simulink model "simpleSM"  (R2021a)
settings: Solver=ode4  StartTime=0.0  StopTime=10.0  FixedStep=1e-4  RelTol=1e-3
settings Model: Creator=compu  LastModifiedBy=compu

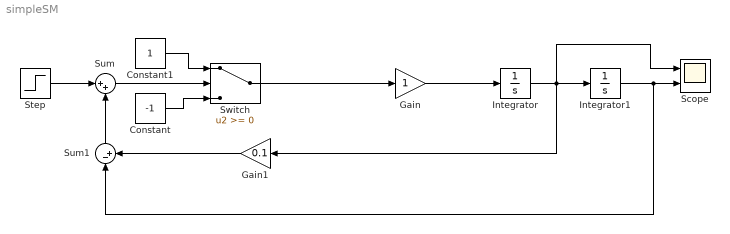
== system simpleSM ==
  Constant : Constant  Value=-1
  Constant1 : Constant
  Gain : Gain
  Gain1 : Gain  Gain=0.1
  Integrator : Integrator
  Integrator1 : Integrator
  Scope : Scope  NumInputPorts=2
  Step : Step  SampleTime=0
  Sum : Sum  Inputs=|++
  Sum1 : Sum  Inputs=|-+
  Switch : Switch  ZeroCross=off
  wires:
  Integrator/1 -> Scope/1, Integrator1/1, Gain1/1
  Switch/1 -> Gain/1
  Gain/1 -> Integrator/1
  Step/1 -> Sum/1
  Sum/1 -> Switch/2
  Integrator1/1 -> Scope/2, Sum1/1
  Sum1/1 -> Sum/2
  Gain1/1 -> Sum1/2
  Constant/1 -> Switch/3
  Constant1/1 -> Switch/1
